simulink model "Inverse_Dynamics_Control_RR_robot_compact"  (R2019b)
settings: Solver=VariableStepAuto  StartTime=0.0  StopTime=20  RelTol=1e-3
settings Model: Creator=manth  LastModifiedBy=manth

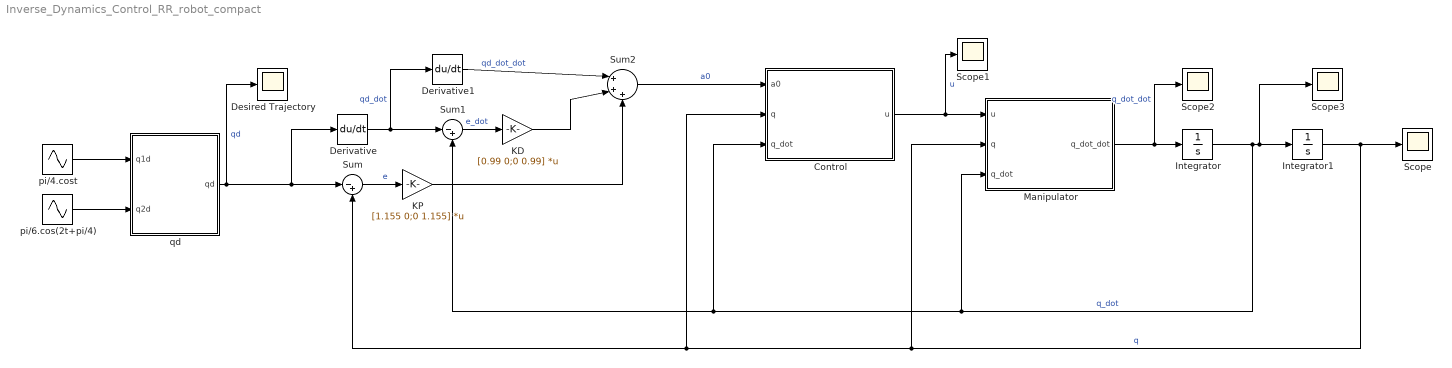
== system Inverse_Dynamics_Control_RR_robot_compact ==
  Control : MATLAB Function  TreatAsAtomicUnit=on
  Derivative : Derivative
  Derivative1 : Derivative
  Desired Trajectory : Scope
  Integrator : Integrator  InitialCondition=[0;0]
  Integrator1 : Integrator  InitialCondition=[0;0]
  KD : Gain  Gain=[0.99 0;0 0.99]  Multiplication=Matrix(K*u) (u vector)
  KP : Gain  Gain=[1.155 0;0 1.155]  Multiplication=Matrix(K*u) (u vector)
  Manipulator : MATLAB Function  TreatAsAtomicUnit=on
  Scope{,1..3} (4 alike) : Scope
  Sum : Sum  Inputs=|-+
  Sum1 : Sum  Inputs=|-+
  Sum2 : Sum  Inputs=|+++
  pi/4.cost : Sin  Amplitude=pi/4  Phase=pi/2  SampleTime=0
  pi/6.cos(2t+pi/4) : Sin  Amplitude=pi/6  Frequency=2  Phase=pi/4  SampleTime=0
  qd : MATLAB Function  TreatAsAtomicUnit=on
  wires:
  pi/4.cost/1 -> qd/1(q1d)
  pi/6.cos(2t+pi/4)/1 -> qd/2(q2d)
  Manipulator/1(q_dot_dot) -> Integrator/1, Scope2/1  "q_dot_dot"
  Integrator/1 -> Scope3/1, Integrator1/1, Sum1/2, Control/3(q_dot), Manipulator/3(q_dot)  "q_dot"
  Integrator1/1 -> Sum/2, Control/2(q), Manipulator/2(q), Scope/1  "q"
  Sum/1 -> KP/1  "e"
  Sum1/1 -> KD/1  "e_dot"
  qd/1(qd) -> Derivative/1, Sum/1, Desired Trajectory/1  "qd"
  Derivative/1 -> Derivative1/1, Sum1/1  "qd_dot"
  Derivative1/1 -> Sum2/1  "qd_dot_dot"
  KD/1 -> Sum2/2
  KP/1 -> Sum2/3
  Sum2/1 -> Control/1(a0)  "a0"
  Control/1(u) -> Scope1/1, Manipulator/1(u)  "u"

== matlab function Inverse_Dynamics_Control_RR_robot_compact/Control ==
  data: a0 input; u output; q input; q_dot input
function u  = Control(a0,q,q_dot)
q1=q(1,1);
q2=q(2,1);
q1_dot=q_dot(1,1);
q2_dot=q_dot(2,1);
m1=0.025;
m2=0.025;
l1=1;
lc1=0.5;
lc2=0.5;
q2=q(2,1);
q1_dot=q_dot(1,1);
q2_dot=q_dot(2,1);
I1=0.0001;
I2=0.0001;
g=9.81;

c11=-m2*l1*lc2*sin(q2)*q2_dot;
c12=-m2*l1*lc2*sin(q2)*(q1_dot+q2_dot);
c21=m2*l1*lc2*(sin(q2))*q1_dot;
c22=0;

C = [c11 c12; c21 c22];

g1= (m1*lc1+m2*l1)*g*cos(q1) + m2*lc2*g*cos(q1+q2);
g2= m2*lc2*g*cos(q1+q2);

G=[g1;g2];

h11= m1*lc1^2 + m2*(l1^2+lc2^2+2*l1*lc2*(cos(q2)))+I1+I2;
h12= m2*(lc2^2 + l1*lc2*(cos(q2)))+ I2;
h21= m2*(lc2^2 + l1*lc2*(cos(q2)))+ I2;
h22= m2*lc2^2 + I2;
H=[h11 h12; h21 h22];
    
u=H*a0+G+C*q_dot;
  
end

== matlab function Inverse_Dynamics_Control_RR_robot_compact/Manipulator ==
  data: u input; q_dot_dot output; q input; q_dot input
function q_dot_dot  = Manipulator(u,q,q_dot)
q1=q(1,1);
q2=q(2,1);
q1_dot=q_dot(1,1);
q2_dot=q_dot(2,1);
m1=0.025;
m2=0.025;
l1=1;
lc1=0.5;
lc2=0.5;
u1 = u(1,1);
u2 = u(2,1);
q2=q(2,1);
q1_dot=q_dot(1,1);
q2_dot=q_dot(2,1);
I1=0.0001;
I2=0.0001;
g=9.81;

c11=-m2*l1*lc2*sin(q2)*q2_dot;
c12=-m2*l1*lc2*sin(q2)*(q1_dot+q2_dot);
c21=m2*l1*lc2*(sin(q2))*q1_dot;
c22=0;

C = [c11 c12; c21 c22];

g1= (m1*lc1+m2*l1)*g*cos(q1) + m2*lc2*g*cos(q1+q2);
g2= m2*lc2*g*cos(q1+q2);

G=[g1;g2];

h11= m1*lc1^2 + m2*(l1^2+lc2^2+2*l1*lc2*(cos(q2)))+I1+I2;
h12= m2*(lc2^2 + l1*lc2*(cos(q2)))+ I2;
h21= m2*(lc2^2 + l1*lc2*(cos(q2)))+ I2;
h22= m2*lc2^2 + I2;
H=[h11 h12; h21 h22];
    
    tou = [u1 u2]';
    tou_1 = C*[q1_dot q2_dot]'+ G;
    
    q_dot_dot = inv(H)\(tou-tou_1);
    
  
end

== matlab function Inverse_Dynamics_Control_RR_robot_compact/qd ==
  data: q1d input; qd output; q2d input
function qd  = qd_calculator(q1d,q2d)

qd=[q1d; q2d];

end
